simulink library "util_fsw_frame_rotation_lib"  (R2015b)
settings: Solver=ode45  SolverMode=SingleTasking  StartTime=0.0  StopTime=10.0  RelTol=1e-3
values from neighbouring files (symbols this model uses):
  de_cos_coeff = [ 1.5419 ... (first row only)    [util_frame_rotation_init.m]
  de_t_poly = fliplr( [66.5392 +0.0130] )    [util_frame_rotation_init.m]
  e10coeff = fliplr([ 15.134 -0.1589763])    [util_frame_rotation_init.m]
  e11coeff = fliplr([119.743 +0.0036096])    [util_frame_rotation_init.m]
  e12coeff = fliplr([239.961 +0.1643573])    [util_frame_rotation_init.m]
  e13coeff = fliplr([ 25.053 +12.9590088])    [util_frame_rotation_init.m]
  e1coeff = fliplr([125.045 -0.0529921])    [util_frame_rotation_init.m]
  e2coeff = fliplr([250.089 -0.1059842])    [util_frame_rotation_init.m]
  e3coeff = fliplr([260.008 +13.0120009])    [util_frame_rotation_init.m]
  e4coeff = fliplr([176.625 +13.3407154])    [util_frame_rotation_init.m]
  e5coeff = fliplr([357.529 +0.9856003])    [util_frame_rotation_init.m]
  e6coeff = fliplr([311.589 +26.4057084])    [util_frame_rotation_init.m]
  e7coeff = fliplr([134.963 +13.0649930])    [util_frame_rotation_init.m]
  e8coeff = fliplr([276.617 +0.3287146])    [util_frame_rotation_init.m]
  e9coeff = fliplr([ 34.226 +1.7484877])    [util_frame_rotation_init.m]
  omega_moon_iau_coeff = [  3.5610 ... (first row only)    [util_frame_rotation_init.m]
  omega_pa_mat_init = [0 0 0; 0 0 0; 0 0 1]    [util_frame_rotation_init.m]
  ra_sin_coeff = [ -3.8787 ... (first row only)    [util_frame_rotation_init.m]
  ra_t_poly = fliplr( [269.9949 +0.0031] )    [util_frame_rotation_init.m]
undefined symbols (not defined in the file or in its folder): central_body_omega_dot, earth_moon_rotation_matrix_select, ini_epoch_seconds, ini_hour, ini_minute, ini_moon_rotation_rate, ini_seconds, kfl_quat_mcmf_to_topo, kfl_target_site_planet_fixed
libraries: util_quat_lib x67, util_common_lib x22, util_info_lib x18, util_fsw_frame_rotation_lib x9, util_extra_lib x1
(part 1 of 2)
settings Model: Creator=Administrator  LastModifiedBy=Mark Agbayani
settings DataIOCC: SaveFormat=Array  SignalLoggingSaveFormat=ModelDataLogs
settings OptimizationCC: BlockReduction=off  BooleanDataType=off  ExpressionDepthLimit=2147483647
settings DebuggingCC: SaveWithParameterizedLinksMsg=none  UnderspecifiedInitializationDetection=Classic  MergeDetectMultiDrivingBlocksExec=none  SignalResolutionControl=TryResolveAllWithWarning  FcnCallInpInsideContextMsg=EnableAllAsWarning  StateNameClashWarn=warning  StrictBusMsg=Warning
settings HardwareCC: ProdBitPerPointer=32  ProdLargestAtomicFloat=None  ProdIntDivRoundTo=Undefined  ProdEndianess=Unspecified  ProdWordSize=32  ProdHWDeviceType=32-bit Generic  TargetUnknown=on
settings GRTTargetCC: GeneratePreprocessorConditionals=Disable all
settings ConfigComp: CovModelRefEnable=Off  CovSFcnEnable=off

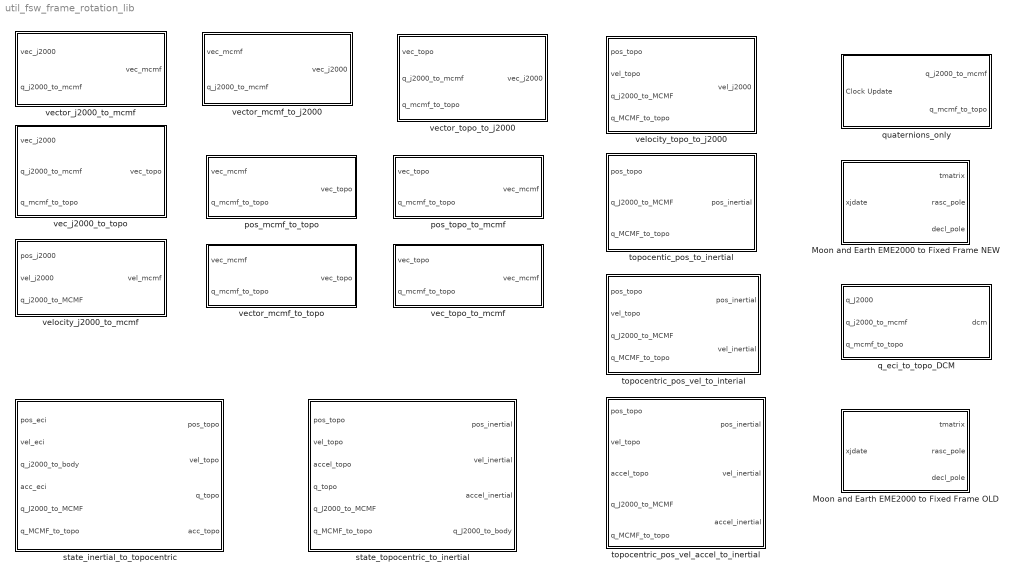
== system util_fsw_frame_rotation_lib ==
  Moon and Earth EME2000 to Fixed Frame NEW : Subsystem
      mask Display:
      | color('blue')
      | text(0.05,0.02,'MoonEx',...
      |  	'HorizontalAlignment','Left',...
      | 	'VerticalAlignment','bottom')
  Moon and Earth EME2000 to Fixed Frame OLD : Subsystem
      mask Display:
      | color('blue')
      | text(0.05,0.02,'MoonEx',...
      |  	'HorizontalAlignment','Left',...
      | 	'VerticalAlignment','bottom')
  pos_mcmf_to_topo : Subsystem
      mask Display:
      | color('blue')
      | text(0.05,0.02,'MoonEx',...
      |  	'HorizontalAlignment','Left',...
      | 	'VerticalAlignment','bottom')
  pos_topo_to_mcmf : Subsystem
      mask Display:
      | color('blue')
      | text(0.05,0.02,'MoonEx',...
      |  	'HorizontalAlignment','Left',...
      | 	'VerticalAlignment','bottom')
  q_eci_to_topo_DCM : Subsystem
      mask Display:
      | color('blue')
      | text(0.05,0.02,'MoonEx',...
      |  	'HorizontalAlignment','Left',...
      | 	'VerticalAlignment','bottom')
  quaternions_only : Subsystem
      mask Display:
      | color('blue')
      | text(0.05,0.02,'MoonEx',...
      |  	'HorizontalAlignment','Left',...
      | 	'VerticalAlignment','bottom')
  state_inertial_to_topocentric : Subsystem
      mask Display:
      | color('blue')
      | text(0.05,0.02,'MoonEx',...
      |  	'HorizontalAlignment','Left',...
      | 	'VerticalAlignment','bottom')
  state_topocentric_to_inertial : Subsystem
      mask Display:
      | color('blue')
      | text(0.05,0.02,'MoonEx',...
      |  	'HorizontalAlignment','Left',...
      | 	'VerticalAlignment','bottom')
  topocentic_pos_to_inertial : Subsystem
      mask Display:
      | color('blue')
      | text(0.05,0.02,'MoonEx',...
      |  	'HorizontalAlignment','Left',...
      | 	'VerticalAlignment','bottom')
  topocentric_pos_vel_accel_to_inertial : Subsystem
      mask Display:
      | color('blue')
      | text(0.05,0.02,'MoonEx',...
      |  	'HorizontalAlignment','Left',...
      | 	'VerticalAlignment','bottom')
  topocentric_pos_vel_to_interial : Subsystem
      mask Display:
      | color('blue')
      | text(0.05,0.02,'MoonEx',...
      |  	'HorizontalAlignment','Left',...
      | 	'VerticalAlignment','bottom')
  vec_j2000_to_topo : Subsystem
      mask Display:
      | color('blue')
      | text(0.05,0.02,'MoonEx',...
      |  	'HorizontalAlignment','Left',...
      | 	'VerticalAlignment','bottom')
  vec_topo_to_mcmf : Subsystem
      mask Display:
      | color('blue')
      | text(0.05,0.02,'MoonEx',...
      |  	'HorizontalAlignment','Left',...
      | 	'VerticalAlignment','bottom')
  vector_j2000_to_mcmf : Subsystem
      mask Display:
      | color('blue')
      | text(0.05,0.02,'MoonEx',...
      |  	'HorizontalAlignment','Left',...
      | 	'VerticalAlignment','bottom')
  vector_mcmf_to_j2000 : Subsystem
      mask Display:
      | color('blue')
      | text(0.05,0.02,'MoonEx',...
      |  	'HorizontalAlignment','Left',...
      | 	'VerticalAlignment','bottom')
  vector_mcmf_to_topo : Subsystem
      mask Display:
      | color('blue')
      | text(0.05,0.02,'MoonEx',...
      |  	'HorizontalAlignment','Left',...
      | 	'VerticalAlignment','bottom')
  vector_topo_to_j2000 : Subsystem
      mask Display:
      | color('blue')
      | text(0.05,0.02,'MoonEx',...
      |  	'HorizontalAlignment','Left',...
      | 	'VerticalAlignment','bottom')
  velocity_j2000_to_mcmf : Subsystem
      mask Display:
      | color('blue')
      | text(0.05,0.02,'MoonEx',...
      |  	'HorizontalAlignment','Left',...
      | 	'VerticalAlignment','bottom')
  velocity_topo_to_j2000 : Subsystem
      mask Display:
      | color('blue')
      | text(0.05,0.02,'MoonEx',...
      |  	'HorizontalAlignment','Left',...
      | 	'VerticalAlignment','bottom')

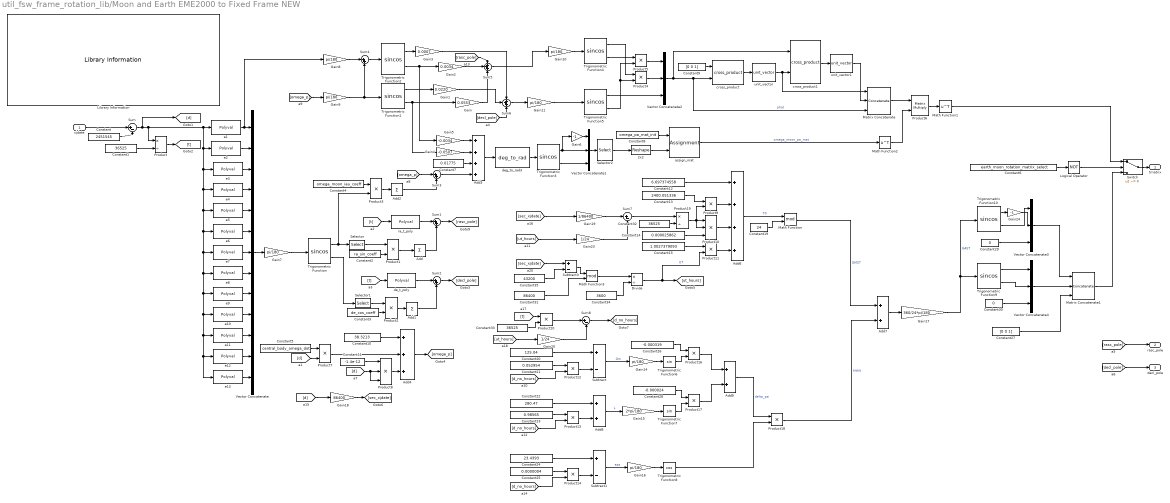
== system util_fsw_frame_rotation_lib/Moon and Earth EME2000 to Fixed Frame NEW ==
  xjdate : Inport
  2x2 : Reshape  OutputDimensionality=Customize  OutputDimensions=[2,2]
  Add : Sum  Inputs=+
  Add1 : Sum  Inputs=+
  Add2 : Sum  Inputs=+
  Add3 : Sum  Inputs=4
  Add4 : Sum  Inputs=3
  Add6 : Sum  Inputs=4
  Add7 : Sum  Inputs=2
  Add8 : Sum  Inputs=2
  Add9 : Sum  Inputs=2
  Constant : Constant  Value=2451545
  Constant1 : Constant  Value=36525
  Constant10 : Constant  Value=38.3213
  Constant11 : Constant  Value=-1.4e-12
  Constant12 : Constant  Value=6.697374558
  Constant13 : Constant  Value=2400.051336
  Constant14 : Constant  Value=0.000025862
  Constant15 : Constant  Value=1.0027379093
  Constant19 : Constant  Value=24
  Constant2 : Constant  Value=ra_sin_coeff
  Constant20 : Constant  Value=125.04
  Constant21 : Constant  Value=0.052954
  Constant22 : Constant  Value=280.47
  Constant23 : Constant  Value=0.98565
  Constant24 : Constant  Value=23.4393
  Constant25 : Constant  Value=0.0000004
  Constant26 : Constant  Value=-0.000319
  Constant27 : Constant  Value=[0 0 1]
  Constant28 : Constant  Value=-0.000024
  Constant29 : Constant  Value=0
  Constant3 : Constant  Value=de_cos_coeff
  Constant30 : Constant  Value=0
  Constant31 : Constant  Value=86400
  Constant32 : Constant  Value=36525
  Constant33 : Constant  Value=36525
  Constant34 : Constant  Value=3600
  Constant35 : Constant  Value=43200
  Constant4 : Constant  Value=omega_moon_iau_coeff
  Constant5 : Constant  Value=central_body_omega_dot
  Constant6 : Constant  Value=earth_moon_rotation_matrix_select
  Constant7 : Constant  Value=0.01775
  Constant8 : Constant  Value=omega_pa_mat_init
  Constant9 : Constant  Value=[0 0 1]
  Divide : Product  Inputs=*/
  Gain : Gain  Gain=0.0553
  Gain1 : Gain  Gain=0.0220
  Gain{7..11,14,16} (7 alike) : Gain  Gain=pi/180
  Gain15 : Gain  Gain=2*pi/180
  Gain17 : Gain  Gain=360/24*pi/180
  Gain18 : Gain  Gain=86400
  Gain19 : Gain  Gain=1/86400
  Gain2 : Gain  Gain=0.0034
  Gain20 : Gain  Gain=1/24
  Gain23 : Gain  Gain=1/24
  Gain24 : Gain  Gain=-1
  Gain3 : Gain  Gain=0.0007
  Gain4 : Gain  Gain=-0.0507
  Gain5 : Gain  Gain=-0.0034
  Gain6 : Gain  Gain=-1
  Library Information : util_info_lib/Library Information  owner='escrane'
  Logical Operator : Logic  Operator=NOT  AllPortsSameDT=off  OutDataTypeStr=boolean
  Math Function : Math  Operator=mod  SaturateOnIntegerOverflow=on
  Math Function1 : Math  Operator=transpose  SaturateOnIntegerOverflow=on
  Math Function2 : Math  Operator=transpose  SaturateOnIntegerOverflow=on
  Math Function3 : Math  Operator=mod  SaturateOnIntegerOverflow=on
  Matrix Concatenate : Concatenate  NumInputs=3  Mode=Multidimensional array  ConcatenateDimension=2
  Matrix Concatenate1 : Concatenate  NumInputs=3  Mode=Multidimensional array  ConcatenateDimension=2
  Product : Product  Inputs=*/
  Product{1..5,7,9,11..14,16..18,20} (15 alike) : Product
  Product10 : Product  Inputs=3
  Product19 : Product  Inputs=*/
  Product6 : Product  Multiplication=Matrix(*)
  Product8 : Product  Inputs=3
  Selector : Selector  InputPortWidth=13  IndexOptions=Index vector (dialog)  Indices=[1 2 3 4 6 10 13]  OutputSizes=1
  Selector1 : Selector  InputPortWidth=13  IndexOptions=Index vector (dialog)  Indices=[1 2 3 4 6 7 10 13]  OutputSizes=1
  Selector2 : Selector  InputPortWidth=3  IndexOptions=Index vector (dialog)  Indices=[3 1 2 3]  OutputSizes=1
  Subtract : Sum  Inputs=+-
  Subtract1 : Sum  Inputs=+-
  Subtract3 : Sum  Inputs=+-
  Sum : Sum  Inputs=|+-
  Sum{1..4} (4 alike) : Sum  Inputs=|++
  Sum5 : Sum  Inputs=+++
  Sum6 : Sum  Inputs=+++
  Sum7 : Sum  Inputs=|+-
  Sum8 : Sum  Inputs=|+-
  Switch : Switch  Criteria=u2 ~= 0
  Trigonometric Function{,1..5,9..10} (8 alike) : Trigonometry  Operator=sincos
  Trigonometric Function6 : Trigonometry
  Trigonometric Function7 : Trigonometry
  Trigonometric Function8 : Trigonometry  Operator=cos
  Vector Concatenate : Concatenate  NumInputs=13
  Vector Concatenate{1..4} (4 alike) : Concatenate  NumInputs=3
  assign_mat : Assignment  NumberOfDimensions=2  IndexOptions=Index vector (dialog),Index vector (dialog)  Indices=[1 2],[1 2]  OutputSizes=1,1
  cross_product : util_common_lib/cross_product  SystemSampleTime=-1
  cross_product1 : util_common_lib/cross_product  SystemSampleTime=-1
  de_t_poly : Polyval  Coefs=de_t_poly
  deg_to_rad3 : util_common_lib/deg_to_rad  SystemSampleTime=-1
  e1 : Polyval  Coefs=e1coeff
  e10 : Polyval  Coefs=e10coeff
  e11 : Polyval  Coefs=e11coeff
  e12 : Polyval  Coefs=e12coeff
  e13 : Polyval  Coefs=e13coeff
  e2 : Polyval  Coefs=e2coeff
  e3 : Polyval  Coefs=e3coeff
  e4 : Polyval  Coefs=e4coeff
  e5 : Polyval  Coefs=e5coeff
  e6 : Polyval  Coefs=e6coeff
  e7 : Polyval  Coefs=e7coeff
  e8 : Polyval  Coefs=e8coeff
  e9 : Polyval  Coefs=e9coeff
  ra_t_poly : Polyval  Coefs=ra_t_poly
  unit_vector : util_common_lib/unit_vector  SystemSampleTime=-1
  unit_vector1 : util_common_lib/unit_vector  SystemSampleTime=-1
  tmatrix : Outport
  rasc_pole : Outport  Port=2
  decl_pole : Outport  Port=3
  wires:
  [sec_xjdate] -> Subtract3/1
  [sec_xjdate] -> Gain19/1
  Subtract3/1 -> Math Function3/1
  Constant35/1 -> Subtract3/2
  Constant34/1 -> Divide/2
  Math Function3/1 -> Divide/1
  Constant31/1 -> Math Function3/2
  Gain18/1 -> [sec_xjdate]
  [d] -> Gain18/1
  Gain24/1 -> Vector Concatenate3/2
  Gain23/1 -> Sum7/2
  Gain19/1 -> Sum7/1
  Sum7/1 -> Product19/1
  [ut_hours] -> Gain23/1
  Sum8/1 -> [d_no_hours]
  Gain20/1 -> Sum8/2
  Product20/1 -> Sum8/1
  [ut_hours] -> Gain20/1
  Constant33/1 -> Product20/2
  [t] -> Product20/1
  [d_no_hours] -> Product12/2
  [d_no_hours] -> Product13/2
  Product19/1 -> Product10/2, Product9/2, Product10/1
  Constant32/1 -> Product19/2
  Vector Concatenate3/1 -> Matrix Concatenate1/1
  Vector Concatenate4/1 -> Matrix Concatenate1/2
  Constant30/1 -> Vector Concatenate4/3
  Trigonometric Function9/2 -> Vector Concatenate4/2
  Trigonometric Function9/1 -> Vector Concatenate4/1
  Constant29/1 -> Vector Concatenate3/3
  Trigonometric Function10/1 -> Gain24/1
  Trigonometric Function10/2 -> Vector Concatenate3/1
  Gain17/1 -> Trigonometric Function9/1, Trigonometric Function10/1  "GAST"
  Constant27/1 -> Matrix Concatenate1/3
  Matrix Concatenate1/1 -> Switch/3
  Add7/1 -> Gain17/1
  Math Function/1 -> Add7/1  "GMST"
  Product18/1 -> Add7/2  "eqeq"
  Trigonometric Function8/1 -> Product18/2
  Add9/1 -> Product18/1  "delta_psi"
  Gain16/1 -> Trigonometric Function8/1
  Subtract1/1 -> Gain16/1  "eps"
  Product17/1 -> Add9/2
  Product16/1 -> Add9/1
  Constant28/1 -> Product17/1
  Trigonometric Function7/1 -> Product17/2
  Gain15/1 -> Trigonometric Function7/1
  Add8/1 -> Gain15/1  "L"
  Trigonometric Function6/1 -> Product16/2
  Constant26/1 -> Product16/1
  Gain14/1 -> Trigonometric Function6/1
  Subtract/1 -> Gain14/1  "Om"
  [d_no_hours] -> Product14/2
  Constant25/1 -> Product14/1
  Product14/1 -> Subtract1/2
  Constant24/1 -> Subtract1/1
  Constant23/1 -> Product13/1
  Product13/1 -> Add8/2
  Constant22/1 -> Add8/1
  Constant21/1 -> Product12/1
  Product12/1 -> Subtract/2
  Constant20/1 -> Subtract/1
  Add6/1 -> Math Function/1  "T0"
  Constant19/1 -> Math Function/2
  Product11/1 -> Add6/4
  Divide/1 -> [ut_hours], Product11/2  "UT"
  Constant15/1 -> Product11/1
  Product10/1 -> Add6/3
  Constant14/1 -> Product10/3
  Product9/1 -> Add6/2
  Constant13/1 -> Product9/1
  Constant12/1 -> Add6/1
  Math Function1/1 -> Switch/1
  Switch/1 -> tmatrix/1
  Logical Operator/1 -> Switch/2
  Constant6/1 -> Logical Operator/1
  [omega_p] -> Sum3/1
  Add4/1 -> [omega_p]
  Product8/1 -> Add4/3
  Product7/1 -> Add4/2
  Constant10/1 -> Add4/1
  [d] -> Product8/2, Product8/3
  Constant11/1 -> Product8/1
  [d] -> Product7/2
  Constant5/1 -> Product7/1
  xjdate/1 -> Sum/1
  Constant/1 -> Sum/2
  Constant1/1 -> Product/2
  Product/1 -> [t]
  Sum/1 -> e10/1, e13/1, e12/1, e11/1, e9/1, e8/1, e7/1, e6/1, e5/1, e4/1, e3/1, e2/1, e1/1, Product/1, [d]
  e1/1 -> Gain8/1, Vector Concatenate/1
  e2/1 -> Vector Concatenate/2
  e3/1 -> Vector Concatenate/3
  e4/1 -> Vector Concatenate/4
  e5/1 -> Vector Concatenate/5
  e6/1 -> Vector Concatenate/6
  e7/1 -> Vector Concatenate/7
  e8/1 -> Vector Concatenate/8
  e9/1 -> Vector Concatenate/9
  e10/1 -> Vector Concatenate/10
  e11/1 -> Vector Concatenate/11
  e12/1 -> Vector Concatenate/12
  e13/1 -> Vector Concatenate/13
  Vector Concatenate/1 -> Gain7/1
  Gain7/1 -> Trigonometric Function/1
  Trigonometric Function/1 -> Product3/2, Selector/1
  Trigonometric Function/2 -> Selector1/1
  [t] -> ra_t_poly/1
  Selector/1 -> Product1/1
  Constant2/1 -> Product1/2
  Product1/1 -> Add/1
  ra_t_poly/1 -> Sum1/1
  Add/1 -> Sum1/2
  Sum1/1 -> [rasc_pole]
  [t] -> de_t_poly/1
  Selector1/1 -> Product2/1
  Constant3/1 -> Product2/2
  Product2/1 -> Add1/1
  de_t_poly/1 -> Sum2/1
  Add1/1 -> Sum2/2
  Sum2/1 -> [decl_pole]
  Constant4/1 -> Product3/1
  Product3/1 -> Add2/1
  Add2/1 -> Sum3/2
  Sum3/1 -> Add3/4
  [omega_p] -> Gain9/1
  Gain9/1 -> Sum4/2, Trigonometric Function1/1
  Gain8/1 -> Sum4/1
  Sum4/1 -> Trigonometric Function2/1
  Trigonometric Function1/2 -> Gain4/1, Gain/1
  Trigonometric Function1/1 -> Gain1/1
  Trigonometric Function2/1 -> Gain3/1
  Trigonometric Function2/2 -> Gain2/1, Gain5/1
  [decl_pole] -> Sum6/3
  [rasc_pole] -> Sum5/1
  Sum5/1 -> Gain10/1
  Sum6/1 -> Gain11/1
  Gain5/1 -> Add3/1
  Gain4/1 -> Add3/2
  Constant7/1 -> Add3/3
  Add3/1 -> deg_to_rad3/1
  deg_to_rad3/1 -> Trigonometric Function3/1
  Trigonometric Function3/2 -> Vector Concatenate1/3
  Trigonometric Function3/1 -> Gain6/1, Vector Concatenate1/2
  Gain6/1 -> Vector Concatenate1/1
  Vector Concatenate1/1 -> Selector2/1
  Selector2/1 -> 2x2/1
  2x2/1 -> assign_mat/2
  Constant8/1 -> assign_mat/1
  assign_mat/1 -> Math Function2/1  "omega_moon_pa_mat"
  Gain10/1 -> Trigonometric Function4/1
  Gain11/1 -> Trigonometric Function5/1
  Trigonometric Function4/1 -> Product4/1
  Trigonometric Function5/1 -> Vector Concatenate2/3
  Trigonometric Function4/2 -> Product5/1
  Product5/1 -> Vector Concatenate2/1
  Product4/1 -> Vector Concatenate2/2
  Vector Concatenate2/1 -> cross_product1/1, Matrix Concatenate/3, cross_product/2  "phat"
  Constant9/1 -> cross_product/1
  cross_product/1 -> unit_vector/1
  unit_vector/1 -> Matrix Concatenate/1, cross_product1/2
  cross_product1/1 -> unit_vector1/1
  unit_vector1/1 -> Matrix Concatenate/2
  Matrix Concatenate/1 -> Product6/1
  Product6/1 -> Math Function1/1
  Gain/1 -> Sum5/3
  Gain2/1 -> Sum5/2
  Gain1/1 -> Sum6/2
  Gain3/1 -> Sum6/1
  Trigonometric Function5/2 -> Product4/2, Product5/2
  Math Function2/1 -> Product6/2
  [rasc_pole] -> rasc_pole/1
  [decl_pole] -> decl_pole/1

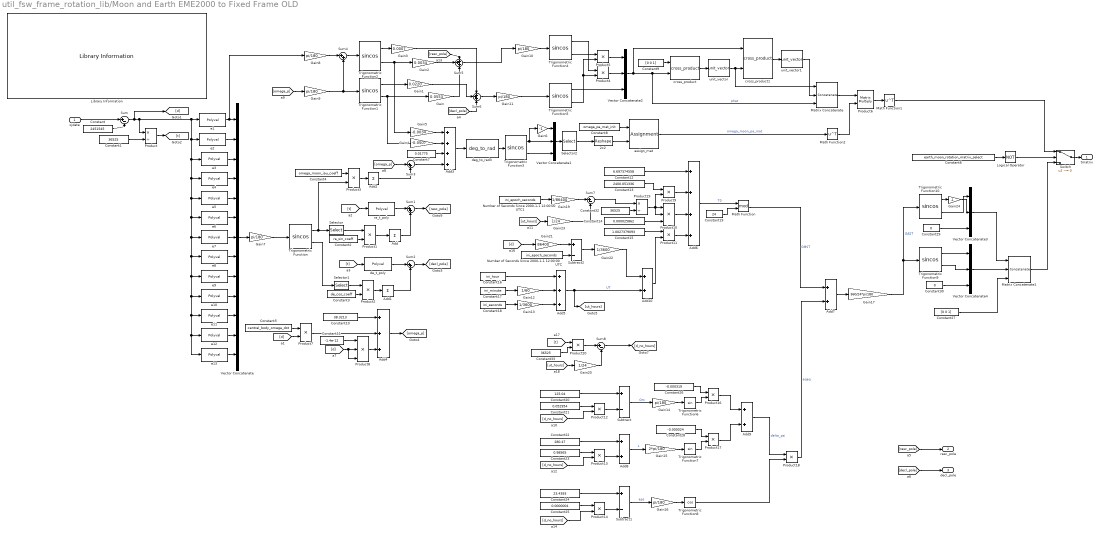
== system util_fsw_frame_rotation_lib/Moon and Earth EME2000 to Fixed Frame OLD ==
  xjdate : Inport
  2x2 : Reshape  OutputDimensionality=Customize  OutputDimensions=[2,2]
  Add : Sum  Inputs=+
  Add1 : Sum  Inputs=+
  Add{7..10} (4 alike) : Sum  Inputs=2
  Add2 : Sum  Inputs=+
  Add3 : Sum  Inputs=4
  Add4 : Sum  Inputs=3
  Add5 : Sum  Inputs=3
  Add6 : Sum  Inputs=4
  Constant : Constant  Value=2451545
  Constant1 : Constant  Value=36525
  Constant10 : Constant  Value=38.3213
  Constant11 : Constant  Value=-1.4e-12
  Constant12 : Constant  Value=6.697374558
  Constant13 : Constant  Value=2400.051336
  Constant14 : Constant  Value=0.000025862
  Constant15 : Constant  Value=1.0027379093
  Constant16 : Constant  Value=ini_hour
  Constant17 : Constant  Value=ini_minute
  Constant18 : Constant  Value=ini_seconds
  Constant19 : Constant  Value=24
  Constant2 : Constant  Value=ra_sin_coeff
  Constant20 : Constant  Value=125.04
  Constant21 : Constant  Value=0.052954
  Constant22 : Constant  Value=280.47
  Constant23 : Constant  Value=0.98565
  Constant24 : Constant  Value=23.4393
  Constant25 : Constant  Value=0.0000004
  Constant26 : Constant  Value=-0.000319
  Constant27 : Constant  Value=[0 0 1]
  Constant28 : Constant  Value=-0.000024
  Constant29 : Constant  Value=0
  Constant3 : Constant  Value=de_cos_coeff
  Constant30 : Constant  Value=0
  Constant32 : Constant  Value=36525
  Constant33 : Constant  Value=36525
  Constant4 : Constant  Value=omega_moon_iau_coeff
  Constant5 : Constant  Value=central_body_omega_dot
  Constant6 : Constant  Value=earth_moon_rotation_matrix_select
  Constant7 : Constant  Value=0.01775
  Constant8 : Constant  Value=omega_pa_mat_init
  Constant9 : Constant  Value=[0 0 1]
  Gain : Gain  Gain=0.0553
  Gain1 : Gain  Gain=0.0220
  Gain{7..11,14,16} (7 alike) : Gain  Gain=pi/180
  Gain12 : Gain  Gain=1/60
  Gain13 : Gain  Gain=1/3600
  Gain15 : Gain  Gain=2*pi/180
  Gain17 : Gain  Gain=360/24*pi/180
  Gain19 : Gain  Gain=1/86400
  Gain2 : Gain  Gain=0.0034
  Gain20 : Gain  Gain=1/24
  Gain21 : Gain  Gain=86400
  Gain22 : Gain  Gain=1/3600
  Gain23 : Gain  Gain=1/24
  Gain24 : Gain  Gain=-1
  Gain3 : Gain  Gain=0.0007
  Gain4 : Gain  Gain=-0.0507
  Gain5 : Gain  Gain=-0.0034
  Gain6 : Gain  Gain=-1
  Library Information : util_info_lib/Library Information  owner='escrane'
  Logical Operator : Logic  Operator=NOT  AllPortsSameDT=off  OutDataTypeStr=boolean
  Math Function : Math  Operator=mod  SaturateOnIntegerOverflow=on
  Math Function1 : Math  Operator=transpose  SaturateOnIntegerOverflow=on
  Math Function2 : Math  Operator=transpose  SaturateOnIntegerOverflow=on
  Matrix Concatenate : Concatenate  NumInputs=3  Mode=Multidimensional array  ConcatenateDimension=2
  Matrix Concatenate1 : Concatenate  NumInputs=3  Mode=Multidimensional array  ConcatenateDimension=2
  Number of Seconds Since 2000-1-1 12:00:00 UTC : Constant  Description=|  Value=ini_epoch_seconds
      | Number of Seconds                   
      | July 4, 2014 22:40:00 UTC           
      | Calculate on Web Site:              
      | www.mbari.org/staff/rich/utccalc.htm
  Number of Seconds Since 2000-1-1 12:00:00 UTC1 : Constant  Description=|  Value=ini_epoch_seconds
      | Number of Seconds                   
      | July 4, 2014 22:40:00 UTC           
      | Calculate on Web Site:              
      | www.mbari.org/staff/rich/utccalc.htm
  Product : Product  Inputs=*/
  Product{1..5,7,9,11..14,16..18,20} (15 alike) : Product
  Product10 : Product  Inputs=3
  Product19 : Product  Inputs=*/
  Product6 : Product  Multiplication=Matrix(*)
  Product8 : Product  Inputs=3
  Selector : Selector  InputPortWidth=13  IndexOptions=Index vector (dialog)  Indices=[1 2 3 4 6 10 13]  OutputSizes=1
  Selector1 : Selector  InputPortWidth=13  IndexOptions=Index vector (dialog)  Indices=[1 2 3 4 6 7 10 13]  OutputSizes=1
  Selector2 : Selector  InputPortWidth=3  IndexOptions=Index vector (dialog)  Indices=[3 1 2 3]  OutputSizes=1
  Subtract : Sum  Inputs=+-
  Subtract1 : Sum  Inputs=+-
  Subtract2 : Sum  Inputs=+-
  Sum : Sum  Inputs=|+-
  Sum{1..4} (4 alike) : Sum  Inputs=|++
  Sum5 : Sum  Inputs=+++
  Sum6 : Sum  Inputs=+++
  Sum7 : Sum  Inputs=|+-
  Sum8 : Sum  Inputs=|+-
  Switch : Switch  Criteria=u2 ~= 0
  Trigonometric Function{,1..5,9..10} (8 alike) : Trigonometry  Operator=sincos
  Trigonometric Function6 : Trigonometry
  Trigonometric Function7 : Trigonometry
  Trigonometric Function8 : Trigonometry  Operator=cos
  Vector Concatenate : Concatenate  NumInputs=13
  Vector Concatenate{1..4} (4 alike) : Concatenate  NumInputs=3
  assign_mat : Assignment  NumberOfDimensions=2  IndexOptions=Index vector (dialog),Index vector (dialog)  Indices=[1 2],[1 2]  OutputSizes=1,1
  cross_product : util_common_lib/cross_product  SystemSampleTime=-1
  cross_product1 : util_common_lib/cross_product  SystemSampleTime=-1
  de_t_poly : Polyval  Coefs=de_t_poly
  deg_to_rad3 : util_common_lib/deg_to_rad  SystemSampleTime=-1
  e1 : Polyval  Coefs=e1coeff
  e10 : Polyval  Coefs=e10coeff
  e11 : Polyval  Coefs=e11coeff
  e12 : Polyval  Coefs=e12coeff
  e13 : Polyval  Coefs=e13coeff
  e2 : Polyval  Coefs=e2coeff
  e3 : Polyval  Coefs=e3coeff
  e4 : Polyval  Coefs=e4coeff
  e5 : Polyval  Coefs=e5coeff
  e6 : Polyval  Coefs=e6coeff
  e7 : Polyval  Coefs=e7coeff
  e8 : Polyval  Coefs=e8coeff
  e9 : Polyval  Coefs=e9coeff
  ra_t_poly : Polyval  Coefs=ra_t_poly
  unit_vector : util_common_lib/unit_vector  SystemSampleTime=-1
  unit_vector1 : util_common_lib/unit_vector  SystemSampleTime=-1
  tmatrix : Outport
  rasc_pole : Outport  Port=2
  decl_pole : Outport  Port=3
  wires:
  [decl_pole] -> decl_pole/1
  [rasc_pole] -> rasc_pole/1
  Math Function2/1 -> Product6/2
  Trigonometric Function5/2 -> Product5/2, Product4/2
  Gain3/1 -> Sum6/1
  Gain1/1 -> Sum6/2
  Gain2/1 -> Sum5/2
  Gain/1 -> Sum5/3
  Product6/1 -> Math Function1/1
  Matrix Concatenate/1 -> Product6/1
  unit_vector1/1 -> Matrix Concatenate/2
  cross_product1/1 -> unit_vector1/1
  unit_vector/1 -> cross_product1/2, Matrix Concatenate/1
  cross_product/1 -> unit_vector/1
  Constant9/1 -> cross_product/1
  Vector Concatenate2/1 -> cross_product/2, Matrix Concatenate/3, cross_product1/1  "phat"
  Product4/1 -> Vector Concatenate2/2
  Product5/1 -> Vector Concatenate2/1
  Trigonometric Function4/2 -> Product5/1
  Trigonometric Function5/1 -> Vector Concatenate2/3
  Trigonometric Function4/1 -> Product4/1
  Gain11/1 -> Trigonometric Function5/1
  Gain10/1 -> Trigonometric Function4/1
  assign_mat/1 -> Math Function2/1  "omega_moon_pa_mat"
  Constant8/1 -> assign_mat/1
  2x2/1 -> assign_mat/2
  Selector2/1 -> 2x2/1
  Vector Concatenate1/1 -> Selector2/1
  Gain6/1 -> Vector Concatenate1/1
  Trigonometric Function3/1 -> Vector Concatenate1/2, Gain6/1
  Trigonometric Function3/2 -> Vector Concatenate1/3
  deg_to_rad3/1 -> Trigonometric Function3/1
  Add3/1 -> deg_to_rad3/1
  Constant7/1 -> Add3/3
  Gain4/1 -> Add3/2
  Gain5/1 -> Add3/1
  Sum6/1 -> Gain11/1
  Sum5/1 -> Gain10/1
  [rasc_pole] -> Sum5/1
  [decl_pole] -> Sum6/3
  Trigonometric Function2/2 -> Gain5/1, Gain2/1
  Trigonometric Function2/1 -> Gain3/1
  Trigonometric Function1/1 -> Gain1/1
  Trigonometric Function1/2 -> Gain/1, Gain4/1
  Sum4/1 -> Trigonometric Function2/1
  Gain8/1 -> Sum4/1
  Gain9/1 -> Trigonometric Function1/1, Sum4/2
  [omega_p] -> Gain9/1
  Sum3/1 -> Add3/4
  Add2/1 -> Sum3/2
  Product3/1 -> Add2/1
  Constant4/1 -> Product3/1
  Sum2/1 -> [decl_pole]
  Add1/1 -> Sum2/2
  de_t_poly/1 -> Sum2/1
  Product2/1 -> Add1/1
  Constant3/1 -> Product2/2
  Selector1/1 -> Product2/1
  [t] -> de_t_poly/1
  Sum1/1 -> [rasc_pole]
  Add/1 -> Sum1/2
  ra_t_poly/1 -> Sum1/1
  Product1/1 -> Add/1
  Constant2/1 -> Product1/2
  Selector/1 -> Product1/1
  [t] -> ra_t_poly/1
  Trigonometric Function/2 -> Selector1/1
  Trigonometric Function/1 -> Selector/1, Product3/2
  Gain7/1 -> Trigonometric Function/1
  Vector Concatenate/1 -> Gain7/1
  e13/1 -> Vector Concatenate/13
  e12/1 -> Vector Concatenate/12
  e11/1 -> Vector Concatenate/11
  e10/1 -> Vector Concatenate/10
  e9/1 -> Vector Concatenate/9
  e8/1 -> Vector Concatenate/8
  e7/1 -> Vector Concatenate/7
  e6/1 -> Vector Concatenate/6
  e5/1 -> Vector Concatenate/5
  e4/1 -> Vector Concatenate/4
  e3/1 -> Vector Concatenate/3
  e2/1 -> Vector Concatenate/2
  e1/1 -> Vector Concatenate/1, Gain8/1
  Sum/1 -> [d], Product/1, e1/1, e2/1, e3/1, e4/1, e5/1, e6/1, e7/1, e8/1, e9/1, e11/1, e12/1, e13/1, e10/1
  Product/1 -> [t]
  Constant1/1 -> Product/2
  Constant/1 -> Sum/2
  xjdate/1 -> Sum/1
  Constant5/1 -> Product7/1
  [d] -> Product7/2
  Constant11/1 -> Product8/1
  [d] -> Product8/3, Product8/2
  Constant10/1 -> Add4/1
  Product7/1 -> Add4/2
  Product8/1 -> Add4/3
  Add4/1 -> [omega_p]
  [omega_p] -> Sum3/1
  Constant6/1 -> Logical Operator/1
  Logical Operator/1 -> Switch/2
  Switch/1 -> tmatrix/1
  Math Function1/1 -> Switch/1
  Constant16/1 -> Add5/1
  Constant18/1 -> Gain13/1
  Constant17/1 -> Gain12/1
  Gain12/1 -> Add5/2
  Gain13/1 -> Add5/3
  Constant12/1 -> Add6/1
  Constant13/1 -> Product9/1
  Product9/1 -> Add6/2
  Constant14/1 -> Product10/3
  Product10/1 -> Add6/3
  Constant15/1 -> Product11/1
  Add5/1 -> Add10/2, [ut_hours]  "UT"
  Product11/1 -> Add6/4
  Constant19/1 -> Math Function/2
  Add6/1 -> Math Function/1  "T0"
  Constant20/1 -> Subtract/1
  Product12/1 -> Subtract/2
  Constant21/1 -> Product12/1
  Constant22/1 -> Add8/1
  Product13/1 -> Add8/2
  Constant23/1 -> Product13/1
  Constant24/1 -> Subtract1/1
  Product14/1 -> Subtract1/2
  Constant25/1 -> Product14/1
  [d_no_hours] -> Product14/2
  Subtract/1 -> Gain14/1  "Om"
  Gain14/1 -> Trigonometric Function6/1
  Constant26/1 -> Product16/1
  Trigonometric Function6/1 -> Product16/2
  Add8/1 -> Gain15/1  "L"
  Gain15/1 -> Trigonometric Function7/1
  Trigonometric Function7/1 -> Product17/2
  Constant28/1 -> Product17/1
  Product16/1 -> Add9/1
  Product17/1 -> Add9/2
  Subtract1/1 -> Gain16/1  "eps"
  Gain16/1 -> Trigonometric Function8/1
  Add9/1 -> Product18/1  "delta_psi"
  Trigonometric Function8/1 -> Product18/2
  Product18/1 -> Add7/2  "eqeq"
  Math Function/1 -> Add7/1  "GMST"
  Add7/1 -> Gain17/1
  Matrix Concatenate1/1 -> Switch/3
  Constant27/1 -> Matrix Concatenate1/3
  Gain17/1 -> Trigonometric Function10/1, Trigonometric Function9/1  "GAST"
  Trigonometric Function10/2 -> Vector Concatenate3/1
  Trigonometric Function10/1 -> Gain24/1
  Constant29/1 -> Vector Concatenate3/3
  Trigonometric Function9/1 -> Vector Concatenate4/1
  Trigonometric Function9/2 -> Vector Concatenate4/2
  Constant30/1 -> Vector Concatenate4/3
  Vector Concatenate4/1 -> Matrix Concatenate1/2
  Vector Concatenate3/1 -> Matrix Concatenate1/1
  Constant32/1 -> Product19/2
  Product19/1 -> Product10/1, Product9/2, Product10/2
  [d_no_hours] -> Product13/2
  [d_no_hours] -> Product12/2
  Add10/1 -> Product11/2
  Gain22/1 -> Add10/1
  [d] -> Gain21/1
  Number of Seconds Since 2000-1-1 12:00:00 UTC/1 -> Subtract2/2
  Gain21/1 -> Subtract2/1
  Subtract2/1 -> Gain22/1
  [t] -> Product20/1
  Constant33/1 -> Product20/2
  [ut_hours] -> Gain20/1
  Product20/1 -> Sum8/1
  Gain20/1 -> Sum8/2
  Sum8/1 -> [d_no_hours]
  Number of Seconds Since 2000-1-1 12:00:00 UTC1/1 -> Gain19/1
  [ut_hours] -> Gain23/1
  Sum7/1 -> Product19/1
  Gain19/1 -> Sum7/1
  Gain23/1 -> Sum7/2
  Gain24/1 -> Vector Concatenate3/2

== system util_fsw_frame_rotation_lib/pos_mcmf_to_topo ==
  vec_mcmf : Inport
  q_mcmf_to_topo : Inport  Port=2
  Constant10 : Constant  Value=kfl_target_site_planet_fixed
  Library Information : util_info_lib/Library Information  owner='NONE'
  Subtract1 : Sum  Inputs=|+-
  quaternion_frame_transformation1 : util_quat_lib/quaternion_frame_transformation  SystemSampleTime=-1
  vec_topo : Outport
  wires:
  [q_mcmf_to_topo] -> quaternion_frame_transformation1/2
  quaternion_frame_transformation1/1 -> vec_topo/1
  q_mcmf_to_topo/1 -> [q_mcmf_to_topo]
  vec_mcmf/1 -> Subtract1/1
  Constant10/1 -> Subtract1/2
  Subtract1/1 -> quaternion_frame_transformation1/1

== system util_fsw_frame_rotation_lib/pos_topo_to_mcmf ==
  vec_topo : Inport
  q_mcmf_to_topo : Inport  Port=2
  Constant10 : Constant  Value=kfl_target_site_planet_fixed
  Library Information : util_info_lib/Library Information  owner='NONE'
  Subtract1 : Sum  Inputs=|++
  quaternion_conjugate q_topo_to_mcmf : util_quat_lib/quaternion_conjugate  SystemSampleTime=-1
  quaternion_frame_transformation v_mcmf : util_quat_lib/quaternion_frame_transformation  SystemSampleTime=-1
  vec_mcmf : Outport
  wires:
  vec_topo/1 -> quaternion_frame_transformation v_mcmf/1
  [q_mcmf_to_topo] -> quaternion_conjugate q_topo_to_mcmf/1
  quaternion_conjugate q_topo_to_mcmf/1 -> quaternion_frame_transformation v_mcmf/2
  Subtract1/1 -> vec_mcmf/1  "Vector MCMF"
  q_mcmf_to_topo/1 -> [q_mcmf_to_topo]
  quaternion_frame_transformation v_mcmf/1 -> Subtract1/1  "Vector MCMF"
  Constant10/1 -> Subtract1/2

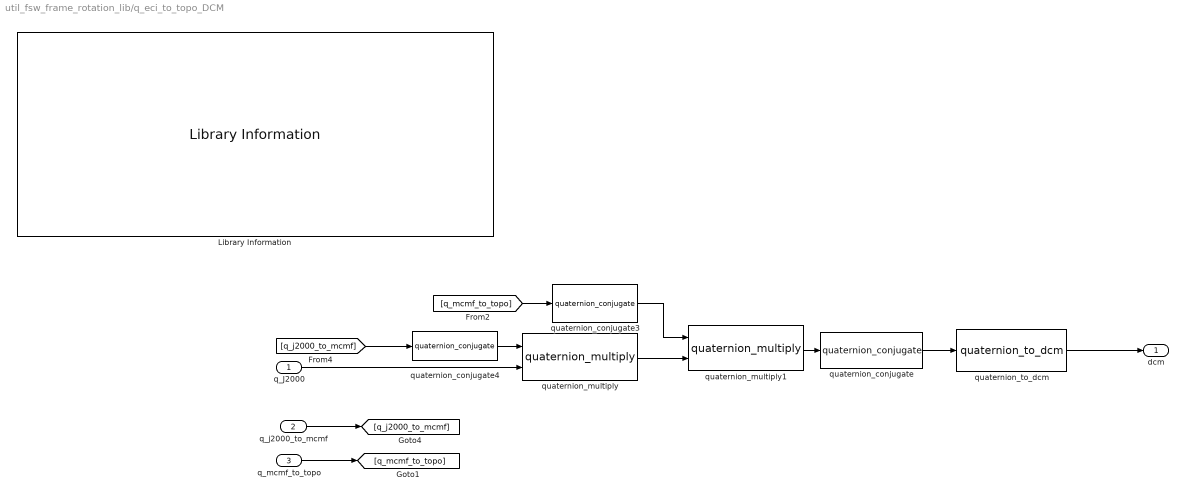
== system util_fsw_frame_rotation_lib/q_eci_to_topo_DCM ==
  q_J2000 : Inport
  q_j2000_to_mcmf : Inport  Port=2
  q_mcmf_to_topo : Inport  Port=3
  Library Information : util_info_lib/Library Information  owner='NONE'
  quaternion_conjugate : util_quat_lib/quaternion_conjugate  SystemSampleTime=-1
  quaternion_conjugate3 : util_quat_lib/quaternion_conjugate  SystemSampleTime=-1
  quaternion_conjugate4 : util_quat_lib/quaternion_conjugate  SystemSampleTime=-1
  quaternion_multiply : util_quat_lib/quaternion_multiply  SystemSampleTime=-1
  quaternion_multiply1 : util_quat_lib/quaternion_multiply  SystemSampleTime=-1
  quaternion_to_dcm : util_quat_lib/quaternion_to_dcm  SystemSampleTime=-1
  dcm : Outport
  wires:
  q_J2000/1 -> quaternion_multiply/2
  quaternion_conjugate4/1 -> quaternion_multiply/1
  quaternion_conjugate3/1 -> quaternion_multiply1/1
  quaternion_multiply/1 -> quaternion_multiply1/2
  quaternion_conjugate/1 -> quaternion_to_dcm/1
  quaternion_multiply1/1 -> quaternion_conjugate/1
  q_mcmf_to_topo/1 -> [q_mcmf_to_topo]
  q_j2000_to_mcmf/1 -> [q_j2000_to_mcmf]
  [q_j2000_to_mcmf] -> quaternion_conjugate4/1
  [q_mcmf_to_topo] -> quaternion_conjugate3/1
  quaternion_to_dcm/1 -> dcm/1

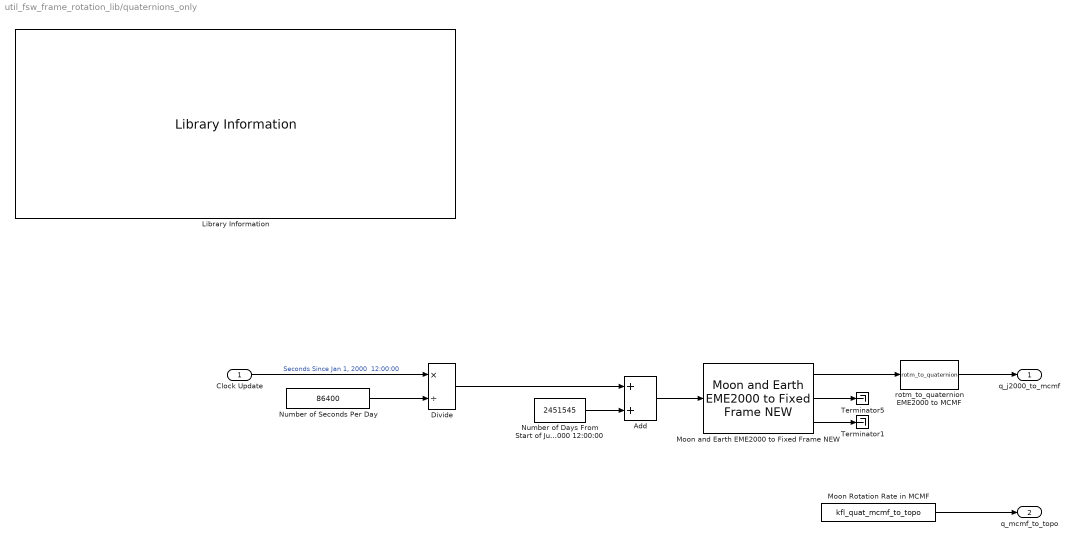
== system util_fsw_frame_rotation_lib/quaternions_only ==
  Clock Update : Inport
  Add : Sum
  Divide : Product  Inputs=*/
  Library Information : util_info_lib/Library Information  owner='NONE'
  Moon Rotation Rate in MCMF : Constant  Value=kfl_quat_mcmf_to_topo
  Moon and Earth EME2000 to Fixed Frame NEW : util_fsw_frame_rotation_lib/Moon and Earth  EME2000 to Fixed Frame NEW  SystemSampleTime=-1
  "Number of Days From Start of Julian Date to Jan 1, 2000 12:00:00" : Constant  Value=2451545
  Number of Seconds Per Day : Constant  Description=|  Value=86400
      | Number of Seconds                   
      | July 4, 2014 22:40:00 UTC           
      | Calculate on Web Site:              
      | www.mbari.org/staff/rich/utccalc.htm
  Terminator1 : Terminator
  Terminator5 : Terminator
  rotm_to_quaternion EME2000 to MCMF : util_extra_lib/rotm_to_quaternion
  q_j2000_to_mcmf : Outport
  q_mcmf_to_topo : Outport  Port=2
  wires:
  Moon Rotation Rate in MCMF/1 -> q_mcmf_to_topo/1
  Divide/1 -> Add/1
  Add/1 -> Moon and Earth EME2000 to Fixed Frame NEW/1
  Moon and Earth EME2000 to Fixed Frame NEW/3 -> Terminator1/1
  Moon and Earth EME2000 to Fixed Frame NEW/2 -> Terminator5/1
  "Number of Days From Start of Julian Date to Jan 1, 2000 12:00:00"/1 -> Add/2
  Clock Update/1 -> Divide/1  "Seconds Since Jan 1, 2000  12:00:00"
  rotm_to_quaternion EME2000 to MCMF/1 -> q_j2000_to_mcmf/1
  Number of Seconds Per Day/1 -> Divide/2
  Moon and Earth EME2000 to Fixed Frame NEW/1 -> rotm_to_quaternion EME2000 to MCMF/1

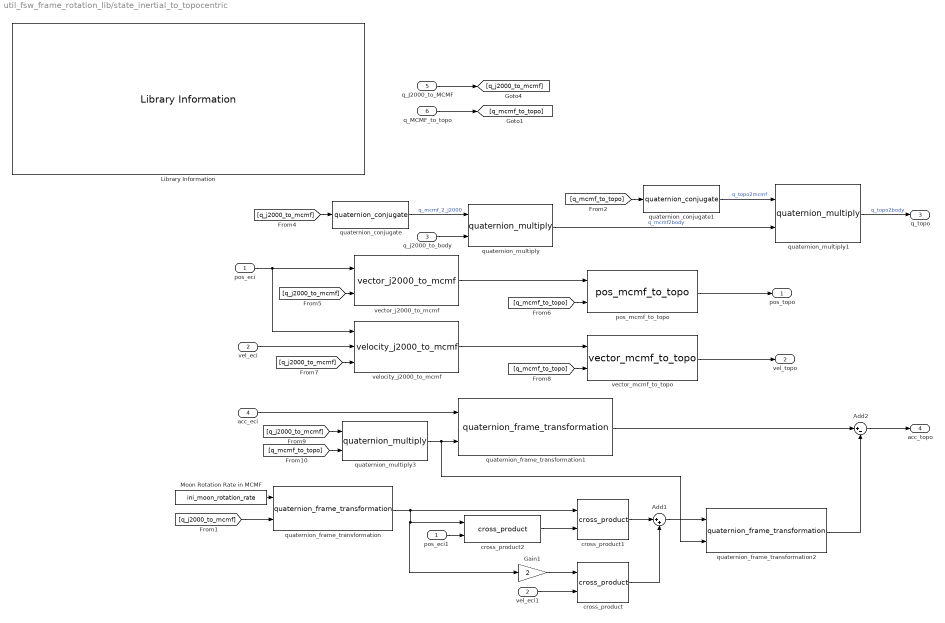
== system util_fsw_frame_rotation_lib/state_inertial_to_topocentric ==
  pos_eci : Inport
  vel_eci : Inport  Port=2
  q_j2000_to_body : Inport  Port=3
  acc_eci : Inport  Port=4
  q_J2000_to_MCMF : Inport  Port=5
  q_MCMF_to_topo : Inport  Port=6
  Add1 : Sum  Inputs=|++
  Add2 : Sum  Inputs=|+-
  Gain1 : Gain  Gain=2
  Library Information : util_info_lib/Library Information  owner='NONE'
  Moon Rotation Rate in MCMF : Constant  Value=ini_moon_rotation_rate
  cross_product : util_common_lib/cross_product  SystemSampleTime=-1
  cross_product1 : util_common_lib/cross_product  SystemSampleTime=-1
  cross_product2 : util_common_lib/cross_product  SystemSampleTime=-1
  pos_eci1 : InportShadow
  pos_mcmf_to_topo : util_fsw_frame_rotation_lib/pos_mcmf_to_topo  SystemSampleTime=-1
  quaternion_conjugate : util_quat_lib/quaternion_conjugate  SystemSampleTime=-1
  quaternion_conjugate1 : util_quat_lib/quaternion_conjugate  SystemSampleTime=-1
  quaternion_frame_transformation : util_quat_lib/quaternion_frame_transformation  SystemSampleTime=-1
  quaternion_frame_transformation1 : util_quat_lib/quaternion_frame_transformation  SystemSampleTime=-1
  quaternion_frame_transformation2 : util_quat_lib/quaternion_frame_transformation  SystemSampleTime=-1
  quaternion_multiply : util_quat_lib/quaternion_multiply  SystemSampleTime=-1
  quaternion_multiply1 : util_quat_lib/quaternion_multiply  SystemSampleTime=-1
  quaternion_multiply3 : util_quat_lib/quaternion_multiply  SystemSampleTime=-1
  vector_j2000_to_mcmf : util_fsw_frame_rotation_lib/vector_j2000_to_mcmf  SystemSampleTime=-1
  vector_mcmf_to_topo : util_fsw_frame_rotation_lib/vector_mcmf_to_topo  SystemSampleTime=-1
  vel_eci1 : InportShadow  Port=2
  velocity_j2000_to_mcmf : util_fsw_frame_rotation_lib/velocity_j2000_to_mcmf  SystemSampleTime=-1
  pos_topo : Outport
  vel_topo : Outport  Port=2
  q_topo : Outport  Port=3
  acc_topo : Outport  Port=4
  wires:
  pos_eci/1 -> velocity_j2000_to_mcmf/1, vector_j2000_to_mcmf/1
  velocity_j2000_to_mcmf/1 -> vector_mcmf_to_topo/1
  pos_mcmf_to_topo/1 -> pos_topo/1
  quaternion_multiply/1 -> quaternion_multiply1/2  "q_mcmf2body"
  quaternion_multiply1/1 -> q_topo/1  "q_topo2body"
  [q_j2000_to_mcmf] -> quaternion_conjugate/1
  quaternion_conjugate/1 -> quaternion_multiply/1  "q_mcmf_2_j2000"
  q_j2000_to_body/1 -> quaternion_multiply/2
  quaternion_conjugate1/1 -> quaternion_multiply1/1  "q_topo2mcmf"
  [q_mcmf_to_topo] -> quaternion_conjugate1/1
  vel_eci/1 -> velocity_j2000_to_mcmf/2
  Add2/1 -> acc_topo/1
  acc_eci/1 -> quaternion_frame_transformation1/1
  quaternion_frame_transformation1/1 -> Add2/1
  cross_product/1 -> Add1/2
  cross_product1/1 -> Add1/1
  pos_eci1/1 -> cross_product2/2
  cross_product2/1 -> cross_product1/2
  vel_eci1/1 -> cross_product/2
  Gain1/1 -> cross_product/1
  quaternion_frame_transformation/1 -> Gain1/1, cross_product2/1, cross_product1/1
  Moon Rotation Rate in MCMF/1 -> quaternion_frame_transformation/1
  [q_j2000_to_mcmf] -> quaternion_frame_transformation/2
  quaternion_multiply3/1 -> quaternion_frame_transformation1/2, quaternion_frame_transformation2/2
  quaternion_frame_transformation2/1 -> Add2/2
  Add1/1 -> quaternion_frame_transformation2/1
  q_MCMF_to_topo/1 -> [q_mcmf_to_topo]
  q_J2000_to_MCMF/1 -> [q_j2000_to_mcmf]
  [q_j2000_to_mcmf] -> vector_j2000_to_mcmf/2
  [q_mcmf_to_topo] -> pos_mcmf_to_topo/2
  [q_j2000_to_mcmf] -> velocity_j2000_to_mcmf/3
  vector_mcmf_to_topo/1 -> vel_topo/1
  [q_mcmf_to_topo] -> vector_mcmf_to_topo/2
  [q_mcmf_to_topo] -> quaternion_multiply3/2
  [q_j2000_to_mcmf] -> quaternion_multiply3/1
  vector_j2000_to_mcmf/1 -> pos_mcmf_to_topo/1

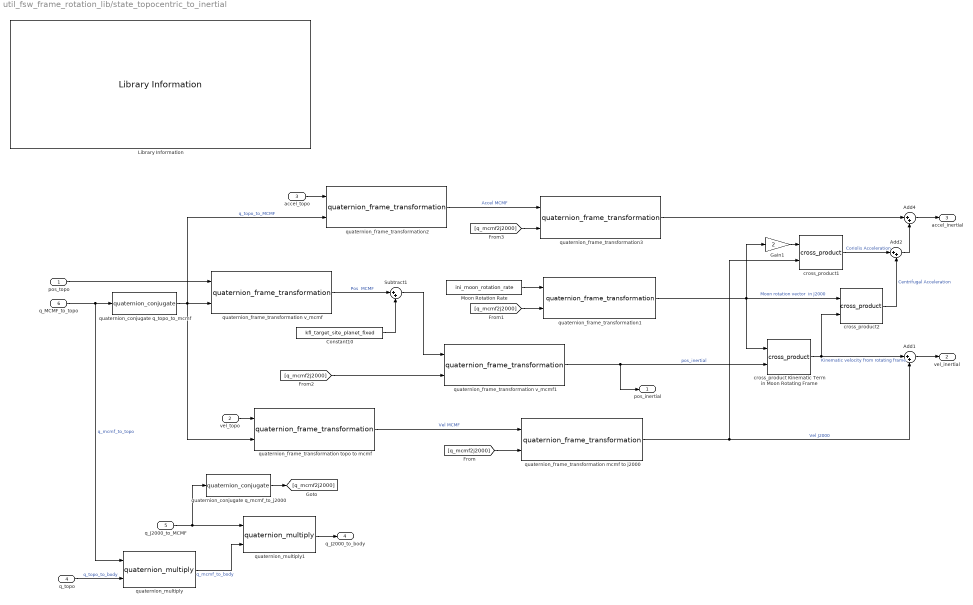
== system util_fsw_frame_rotation_lib/state_topocentric_to_inertial ==
  pos_topo : Inport
  vel_topo : Inport  Port=2
  accel_topo : Inport  Port=3
  q_topo : Inport  Port=4
  q_J2000_to_MCMF : Inport  Port=5
  q_MCMF_to_topo : Inport  Port=6
  Add1 : Sum  Inputs=|++
  Add2 : Sum  Inputs=|++
  Add4 : Sum  Inputs=|++
  Constant10 : Constant  Value=kfl_target_site_planet_fixed
  Gain1 : Gain  Gain=2
  Library Information : util_info_lib/Library Information  owner='NONE'
  Moon Rotation Rate : Constant  Value=ini_moon_rotation_rate
  Subtract1 : Sum  Inputs=|++
  cross_product Kinematic Term in Moon Rotating Frame : util_common_lib/cross_product  SystemSampleTime=-1
  cross_product1 : util_common_lib/cross_product  SystemSampleTime=-1
  cross_product2 : util_common_lib/cross_product  SystemSampleTime=-1
  quaternion_conjugate q_mcmf_to_j2000 : util_quat_lib/quaternion_conjugate  SystemSampleTime=-1
  quaternion_conjugate q_topo_to_mcmf : util_quat_lib/quaternion_conjugate  SystemSampleTime=-1
  quaternion_frame_transformation mcmf to j2000 : util_quat_lib/quaternion_frame_transformation  SystemSampleTime=-1
  quaternion_frame_transformation topo to mcmf : util_quat_lib/quaternion_frame_transformation  SystemSampleTime=-1
  quaternion_frame_transformation v_mcmf : util_quat_lib/quaternion_frame_transformation  SystemSampleTime=-1
  quaternion_frame_transformation v_mcmf1 : util_quat_lib/quaternion_frame_transformation  SystemSampleTime=-1
  quaternion_frame_transformation1 : util_quat_lib/quaternion_frame_transformation  SystemSampleTime=-1
  quaternion_frame_transformation2 : util_quat_lib/quaternion_frame_transformation  SystemSampleTime=-1
  quaternion_frame_transformation3 : util_quat_lib/quaternion_frame_transformation  SystemSampleTime=-1
  quaternion_multiply : util_quat_lib/quaternion_multiply  SystemSampleTime=-1
  quaternion_multiply1 : util_quat_lib/quaternion_multiply  SystemSampleTime=-1
  pos_inertial : Outport
  vel_inertial : Outport  Port=2
  accel_inertial : Outport  Port=3
  q_J2000_to_body : Outport  Port=4
  wires:
  cross_product2/1 -> Add2/2  "Centrifugal Acceleration"
  Add4/1 -> accel_inertial/1
  Add2/1 -> Add4/2
  cross_product1/1 -> Add2/1  "Coriolis Acceleration"
  Gain1/1 -> cross_product1/1
  quaternion_frame_transformation3/1 -> Add4/1
  accel_topo/1 -> quaternion_frame_transformation2/1
  [q_mcmf2j2000] -> quaternion_frame_transformation3/2
  quaternion_frame_transformation2/1 -> quaternion_frame_transformation3/1  "Accel MCMF"
  Constant10/1 -> Subtract1/2
  quaternion_frame_transformation v_mcmf/1 -> Subtract1/1  "Pos  MCMF"
  quaternion_frame_transformation v_mcmf1/1 -> cross_product Kinematic Term in Moon Rotating Frame/2, pos_inertial/1  "pos_inertial"
  [q_mcmf2j2000] -> quaternion_frame_transformation v_mcmf1/2
  quaternion_conjugate q_mcmf_to_j2000/1 -> [q_mcmf2j2000]
  [q_mcmf2j2000] -> quaternion_frame_transformation mcmf to j2000/2
  cross_product Kinematic Term in Moon Rotating Frame/1 -> cross_product2/2, Add1/1  "Kinematic velocity from rotating frame"
  quaternion_frame_transformation mcmf to j2000/1 -> Add1/2, cross_product1/2  "Vel J2000"
  Add1/1 -> vel_inertial/1
  quaternion_frame_transformation1/1 -> Gain1/1, cross_product2/1, cross_product Kinematic Term in Moon Rotating Frame/1  "Moon rotation vector  in J2000"
  Moon Rotation Rate/1 -> quaternion_frame_transformation1/1
  quaternion_frame_transformation topo to mcmf/1 -> quaternion_frame_transformation mcmf to j2000/1  "Vel MCMF"
  vel_topo/1 -> quaternion_frame_transformation topo to mcmf/1
  Subtract1/1 -> quaternion_frame_transformation v_mcmf1/1
  [q_mcmf2j2000] -> quaternion_frame_transformation1/2
  quaternion_conjugate q_topo_to_mcmf/1 -> quaternion_frame_transformation v_mcmf/2, quaternion_frame_transformation2/2, quaternion_frame_transformation topo to mcmf/2  "q_topo_to_MCMF"
  pos_topo/1 -> quaternion_frame_transformation v_mcmf/1
  q_topo/1 -> quaternion_multiply/2  "q_topo_to_body"
  q_MCMF_to_topo/1 -> quaternion_multiply/1, quaternion_conjugate q_topo_to_mcmf/1  "q_mcmf_to_topo"
  quaternion_multiply/1 -> quaternion_multiply1/2  "q_mcmf_to_body"
  q_J2000_to_MCMF/1 -> quaternion_conjugate q_mcmf_to_j2000/1, quaternion_multiply1/1
  quaternion_multiply1/1 -> q_J2000_to_body/1

== system util_fsw_frame_rotation_lib/topocentic_pos_to_inertial ==
  pos_topo : Inport
  q_J2000_to_MCMF : Inport  Port=2
  q_MCMF_to_topo : Inport  Port=3
  Constant10 : Constant  Value=kfl_target_site_planet_fixed
  Library Information : util_info_lib/Library Information  owner='NONE'
  Subtract1 : Sum  Inputs=|++
  quaternion_conjugate q_mcmf_to_j2000 : util_quat_lib/quaternion_conjugate  SystemSampleTime=-1
  quaternion_conjugate q_topo_to_mcmf : util_quat_lib/quaternion_conjugate  SystemSampleTime=-1
  quaternion_frame_transformation v_mcmf : util_quat_lib/quaternion_frame_transformation  SystemSampleTime=-1
  quaternion_frame_transformation v_mcmf1 : util_quat_lib/quaternion_frame_transformation  SystemSampleTime=-1
  pos_inertial : Outport
  wires:
  Constant10/1 -> Subtract1/2
  quaternion_frame_transformation v_mcmf/1 -> Subtract1/1  "Pos  MCMF"
  quaternion_frame_transformation v_mcmf1/1 -> pos_inertial/1  "pos_inertial"
  quaternion_conjugate q_mcmf_to_j2000/1 -> quaternion_frame_transformation v_mcmf1/2
  q_J2000_to_MCMF/1 -> quaternion_conjugate q_mcmf_to_j2000/1
  Subtract1/1 -> quaternion_frame_transformation v_mcmf1/1  "Pos  MCMF"
  quaternion_conjugate q_topo_to_mcmf/1 -> quaternion_frame_transformation v_mcmf/2
  q_MCMF_to_topo/1 -> quaternion_conjugate q_topo_to_mcmf/1
  pos_topo/1 -> quaternion_frame_transformation v_mcmf/1

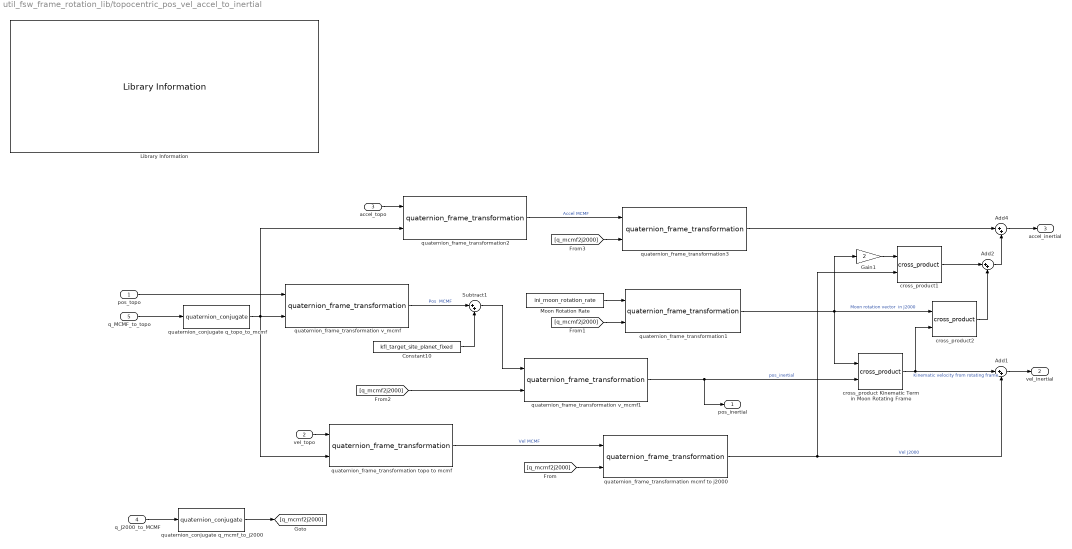
== system util_fsw_frame_rotation_lib/topocentric_pos_vel_accel_to_inertial ==
  pos_topo : Inport
  vel_topo : Inport  Port=2
  accel_topo : Inport  Port=3
  q_J2000_to_MCMF : Inport  Port=4
  q_MCMF_to_topo : Inport  Port=5
  Add1 : Sum  Inputs=|++
  Add2 : Sum  Inputs=|++
  Add4 : Sum  Inputs=|++
  Constant10 : Constant  Value=kfl_target_site_planet_fixed
  Gain1 : Gain  Gain=2
  Library Information : util_info_lib/Library Information  owner='NONE'
  Moon Rotation Rate : Constant  Value=ini_moon_rotation_rate
  Subtract1 : Sum  Inputs=|++
  cross_product Kinematic Term in Moon Rotating Frame : util_common_lib/cross_product  SystemSampleTime=-1
  cross_product1 : util_common_lib/cross_product  SystemSampleTime=-1
  cross_product2 : util_common_lib/cross_product  SystemSampleTime=-1
  quaternion_conjugate q_mcmf_to_j2000 : util_quat_lib/quaternion_conjugate  SystemSampleTime=-1
  quaternion_conjugate q_topo_to_mcmf : util_quat_lib/quaternion_conjugate  SystemSampleTime=-1
  quaternion_frame_transformation mcmf to j2000 : util_quat_lib/quaternion_frame_transformation  SystemSampleTime=-1
  quaternion_frame_transformation topo to mcmf : util_quat_lib/quaternion_frame_transformation  SystemSampleTime=-1
  quaternion_frame_transformation v_mcmf : util_quat_lib/quaternion_frame_transformation  SystemSampleTime=-1
  quaternion_frame_transformation v_mcmf1 : util_quat_lib/quaternion_frame_transformation  SystemSampleTime=-1
  quaternion_frame_transformation1 : util_quat_lib/quaternion_frame_transformation  SystemSampleTime=-1
  quaternion_frame_transformation2 : util_quat_lib/quaternion_frame_transformation  SystemSampleTime=-1
  quaternion_frame_transformation3 : util_quat_lib/quaternion_frame_transformation  SystemSampleTime=-1
  pos_inertial : Outport
  vel_inertial : Outport  Port=2
  accel_inertial : Outport  Port=3
  wires:
  pos_topo/1 -> quaternion_frame_transformation v_mcmf/1
  q_MCMF_to_topo/1 -> quaternion_conjugate q_topo_to_mcmf/1
  quaternion_conjugate q_topo_to_mcmf/1 -> quaternion_frame_transformation topo to mcmf/2, quaternion_frame_transformation2/2, quaternion_frame_transformation v_mcmf/2
  [q_mcmf2j2000] -> quaternion_frame_transformation1/2
  Subtract1/1 -> quaternion_frame_transformation v_mcmf1/1
  vel_topo/1 -> quaternion_frame_transformation topo to mcmf/1
  quaternion_frame_transformation topo to mcmf/1 -> quaternion_frame_transformation mcmf to j2000/1  "Vel MCMF"
  Moon Rotation Rate/1 -> quaternion_frame_transformation1/1
  quaternion_frame_transformation1/1 -> cross_product Kinematic Term in Moon Rotating Frame/1, cross_product2/1, Gain1/1  "Moon rotation vector  in J2000"
  Add1/1 -> vel_inertial/1
  quaternion_frame_transformation mcmf to j2000/1 -> cross_product1/2, Add1/2  "Vel J2000"
  cross_product Kinematic Term in Moon Rotating Frame/1 -> Add1/1, cross_product2/2  "Kinematic velocity from rotating frame"
  [q_mcmf2j2000] -> quaternion_frame_transformation mcmf to j2000/2
  q_J2000_to_MCMF/1 -> quaternion_conjugate q_mcmf_to_j2000/1
  quaternion_conjugate q_mcmf_to_j2000/1 -> [q_mcmf2j2000]
  [q_mcmf2j2000] -> quaternion_frame_transformation v_mcmf1/2
  quaternion_frame_transformation v_mcmf1/1 -> pos_inertial/1, cross_product Kinematic Term in Moon Rotating Frame/2  "pos_inertial"
  quaternion_frame_transformation v_mcmf/1 -> Subtract1/1  "Pos  MCMF"
  Constant10/1 -> Subtract1/2
  quaternion_frame_transformation2/1 -> quaternion_frame_transformation3/1  "Accel MCMF"
  [q_mcmf2j2000] -> quaternion_frame_transformation3/2
  accel_topo/1 -> quaternion_frame_transformation2/1
  quaternion_frame_transformation3/1 -> Add4/1
  Gain1/1 -> cross_product1/1
  cross_product1/1 -> Add2/1
  Add2/1 -> Add4/2
  Add4/1 -> accel_inertial/1
  cross_product2/1 -> Add2/2

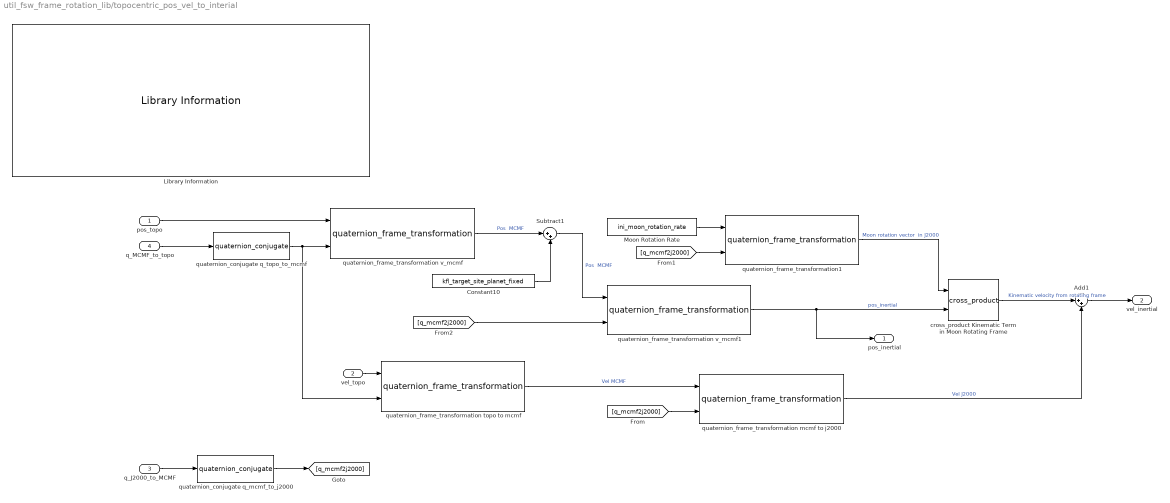
== system util_fsw_frame_rotation_lib/topocentric_pos_vel_to_interial ==
  pos_topo : Inport
  vel_topo : Inport  Port=2
  q_J2000_to_MCMF : Inport  Port=3
  q_MCMF_to_topo : Inport  Port=4
  Add1 : Sum  Inputs=|++
  Constant10 : Constant  Value=kfl_target_site_planet_fixed
  Library Information : util_info_lib/Library Information  owner='NONE'
  Moon Rotation Rate : Constant  Value=ini_moon_rotation_rate
  Subtract1 : Sum  Inputs=|++
  cross_product Kinematic Term in Moon Rotating Frame : util_common_lib/cross_product  SystemSampleTime=-1
  quaternion_conjugate q_mcmf_to_j2000 : util_quat_lib/quaternion_conjugate  SystemSampleTime=-1
  quaternion_conjugate q_topo_to_mcmf : util_quat_lib/quaternion_conjugate  SystemSampleTime=-1
  quaternion_frame_transformation mcmf to j2000 : util_quat_lib/quaternion_frame_transformation  SystemSampleTime=-1
  quaternion_frame_transformation topo to mcmf : util_quat_lib/quaternion_frame_transformation  SystemSampleTime=-1
  quaternion_frame_transformation v_mcmf : util_quat_lib/quaternion_frame_transformation  SystemSampleTime=-1
  quaternion_frame_transformation v_mcmf1 : util_quat_lib/quaternion_frame_transformation  SystemSampleTime=-1
  quaternion_frame_transformation1 : util_quat_lib/quaternion_frame_transformation  SystemSampleTime=-1
  pos_inertial : Outport
  vel_inertial : Outport  Port=2
  wires:
  pos_topo/1 -> quaternion_frame_transformation v_mcmf/1
  q_MCMF_to_topo/1 -> quaternion_conjugate q_topo_to_mcmf/1
  quaternion_conjugate q_topo_to_mcmf/1 -> quaternion_frame_transformation topo to mcmf/2, quaternion_frame_transformation v_mcmf/2
  [q_mcmf2j2000] -> quaternion_frame_transformation1/2
  Subtract1/1 -> quaternion_frame_transformation v_mcmf1/1  "Pos  MCMF"
  vel_topo/1 -> quaternion_frame_transformation topo to mcmf/1
  quaternion_frame_transformation topo to mcmf/1 -> quaternion_frame_transformation mcmf to j2000/1  "Vel MCMF"
  Moon Rotation Rate/1 -> quaternion_frame_transformation1/1
  quaternion_frame_transformation1/1 -> cross_product Kinematic Term in Moon Rotating Frame/1  "Moon rotation vector  in J2000"
  Add1/1 -> vel_inertial/1
  quaternion_frame_transformation mcmf to j2000/1 -> Add1/2  "Vel J2000"
  cross_product Kinematic Term in Moon Rotating Frame/1 -> Add1/1  "Kinematic velocity from rotating frame"
  [q_mcmf2j2000] -> quaternion_frame_transformation mcmf to j2000/2
  q_J2000_to_MCMF/1 -> quaternion_conjugate q_mcmf_to_j2000/1
  quaternion_conjugate q_mcmf_to_j2000/1 -> [q_mcmf2j2000]
  [q_mcmf2j2000] -> quaternion_frame_transformation v_mcmf1/2
  quaternion_frame_transformation v_mcmf1/1 -> pos_inertial/1, cross_product Kinematic Term in Moon Rotating Frame/2  "pos_inertial"
  quaternion_frame_transformation v_mcmf/1 -> Subtract1/1  "Pos  MCMF"
  Constant10/1 -> Subtract1/2

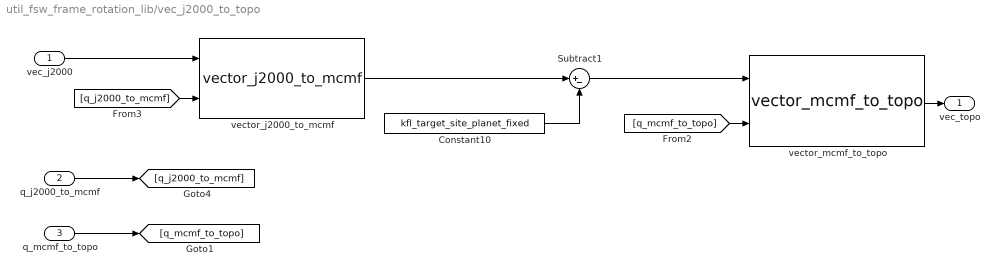
== system util_fsw_frame_rotation_lib/vec_j2000_to_topo ==
  vec_j2000 : Inport
  q_j2000_to_mcmf : Inport  Port=2
  q_mcmf_to_topo : Inport  Port=3
  Constant10 : Constant  Value=kfl_target_site_planet_fixed
  Subtract1 : Sum  Inputs=|+-
  vector_j2000_to_mcmf : util_fsw_frame_rotation_lib/vector_j2000_to_mcmf  SystemSampleTime=-1
  vector_mcmf_to_topo : util_fsw_frame_rotation_lib/vector_mcmf_to_topo  SystemSampleTime=-1
  vec_topo : Outport
  wires:
  vector_mcmf_to_topo/1 -> vec_topo/1
  q_mcmf_to_topo/1 -> [q_mcmf_to_topo]
  q_j2000_to_mcmf/1 -> [q_j2000_to_mcmf]
  vec_j2000/1 -> vector_j2000_to_mcmf/1
  [q_j2000_to_mcmf] -> vector_j2000_to_mcmf/2
  [q_mcmf_to_topo] -> vector_mcmf_to_topo/2
  vector_j2000_to_mcmf/1 -> Subtract1/1
  Subtract1/1 -> vector_mcmf_to_topo/1
  Constant10/1 -> Subtract1/2
